simulink model "AW_test_bachup"  (R2015a)
settings: Solver=ode5  StartTime=0.0  StopTime=0.5  FixedStep=1e-5  MaxStep=5e-5  MinStep=1e-14  RelTol=1e-12  AbsTol=1e-12
values from neighbouring files (symbols this model uses):
  Ak = [-672.634870495 -2626.58972998 -46.1193303275 25.5793500122 108.891317034 -102.718752792 -245.794654799 -577.315326704 39.8827087547 153.58157137 60.36854216 -207.81122515 ... (144 elements, 12x12)]    [controller.mat]    (also in main_matlab.m = rlqg.A)
  Bk = [0.204306341627 1.11161335273 -0.324978673641 2.85402340631 -4.5813117605 2.97328839236 -0.174709893359 1.31662160979 2.94898293865 13.5567055967 -0.791381118401 0.0552385579013]    [controller.mat]    (also in main_matlab.m = rlqg.B)
  Ck = [534.788956442 909.016401092 107.069958755 -410.092366717 -1097.26369634 478.53061829 -894.210554118 460.341899649 -450.064931583 371.993181033 532.787728171 55.8162878584 ... (24 elements, 2x12)]    [controller.mat]    (also in main_matlab.m = rlqg.C)
  Dk = [0 0]    [controller.mat]    (also in main_matlab.m = rlqg.D)
  dumsys1 = ss(Ap+Bp*F,Bp*E,F,E-eye(size(E)))    [main_matlab.m]
  dumsys2 = ss(Ap+Bp*F,Bp*E,Cp+Dp*F,Dp*E)    [main_matlab.m]
undefined symbols (not defined in the file or in its folder): Af, Bf, Cf, Hf
settings Model: Creator=p4wp4w  LastModifiedBy=Ablah

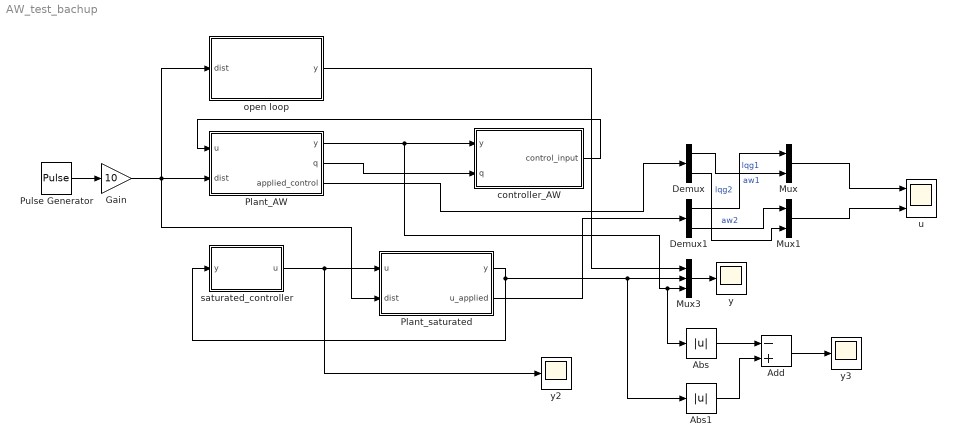
== system AW_test_bachup ==
  Abs : Abs
  Abs1 : Abs
  Add : Sum  Inputs=-+
  Demux : Demux  Outputs=2
  Demux1 : Demux  Outputs=2
  Gain : Gain  Gain=10
  Mux : Mux  Inputs=2
  Mux1 : Mux  Inputs=2
  Mux3 : Mux  Inputs=3
  Plant_AW : Subsystem
  Plant_saturated : Subsystem
  Pulse Generator : DiscretePulseGenerator  PulseType=Time based  Period=0.5  PulseWidth=10
  controller_AW : Subsystem
  open loop : Subsystem
  "saturated_controller " : Subsystem
  u : Scope  NumInputPorts=2
      settings: ShowLegends=on  YMin=-0.45~-0.2  YMax=0.2~0.125
  y : Scope
      settings: ShowLegends=on
  y2 : Scope
      settings: SaveName=ScopeData6
  y3 : Scope
      settings: ShowLegends=on  SaveName=ScopeData3
  wires:
  Plant_AW/1(y) -> Abs/1, Mux3/3, controller_AW/1(y)
  controller_AW/1("control_input ") -> Plant_AW/1(u)
  Pulse Generator/1 -> Gain/1
  Plant_saturated/1(y) -> Abs1/1, Mux3/2, "saturated_controller "/1(y)
  Demux1/1 -> Mux/1  "aw1"
  Demux/1 -> Mux/2  "lqg1"
  Demux1/2 -> Mux1/1  "aw2"
  Demux/2 -> Mux1/2  "lqg2"
  Mux/1 -> u/1
  Mux1/1 -> u/2
  Plant_saturated/2(u_applied) -> Demux1/1
  Gain/1 -> Plant_saturated/2(dist), open loop/1(dist), Plant_AW/2(dist)
  open loop/1(y) -> Mux3/1
  Mux3/1 -> y/1
  "saturated_controller "/1(u) -> y2/1, Plant_saturated/1(u)
  Abs/1 -> Add/1
  Abs1/1 -> Add/2
  Add/1 -> y3/1
  Plant_AW/2(q) -> controller_AW/2(q)
  Plant_AW/3(applied_control) -> Demux/1

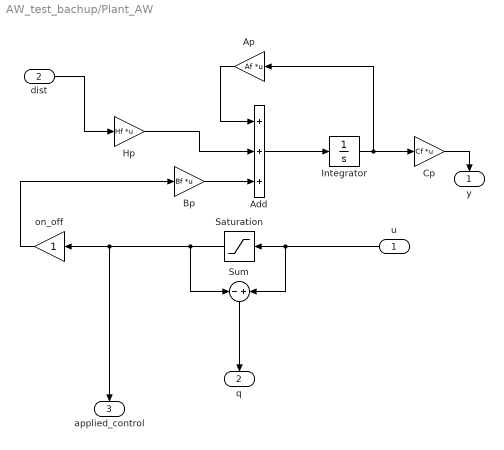
== system AW_test_bachup/Plant_AW ==
  u : Inport
  dist : Inport  Port=2
  Add : Sum  Inputs=+++
  Ap : Gain  Gain=Af  Multiplication=Matrix(K*u)
  Bp : Gain  Gain=Bf  Multiplication=Matrix(K*u)
  Cp : Gain  Gain=Cf  Multiplication=Matrix(K*u)
  Hp : Gain  Gain=Hf  Multiplication=Matrix(K*u)
  Integrator : Integrator
  Saturation : Saturate  UpperLimit=2  LowerLimit=-2
  Sum : Sum  Inputs=-|+
  on_off : Gain
  y : Outport
  q : Outport  Port=2
  applied_control : Outport  Port=3
  wires:
  Add/1 -> Integrator/1
  Cp/1 -> y/1
  Hp/1 -> Add/2
  on_off/1 -> Bp/1
  Integrator/1 -> Cp/1, Ap/1
  Ap/1 -> Add/1
  Bp/1 -> Add/3
  dist/1 -> Hp/1
  u/1 -> Sum/2, Saturation/1
  Saturation/1 -> Sum/1, on_off/1, applied_control/1
  Sum/1 -> q/1

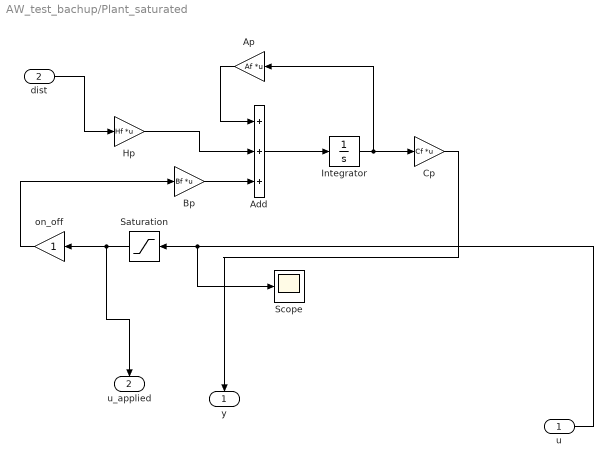
== system AW_test_bachup/Plant_saturated ==
  u : Inport
  dist : Inport  Port=2
  Add : Sum  Inputs=+++
  Ap : Gain  Gain=Af  Multiplication=Matrix(K*u)
  Bp : Gain  Gain=Bf  Multiplication=Matrix(K*u)
  Cp : Gain  Gain=Cf  Multiplication=Matrix(K*u)
  Hp : Gain  Gain=Hf  Multiplication=Matrix(K*u)
  Integrator : Integrator
  Saturation : Saturate  UpperLimit=2  LowerLimit=-2
  Scope : Scope
      settings: YMin=-10  YMax=10  SaveName=ScopeData2
  on_off : Gain
  y : Outport
  u_applied : Outport  Port=2
  wires:
  dist/1 -> Hp/1
  Bp/1 -> Add/3
  u/1 -> Scope/1, Saturation/1
  Ap/1 -> Add/1
  Saturation/1 -> u_applied/1, on_off/1
  Integrator/1 -> Ap/1, Cp/1
  on_off/1 -> Bp/1
  Hp/1 -> Add/2
  Cp/1 -> y/1
  Add/1 -> Integrator/1

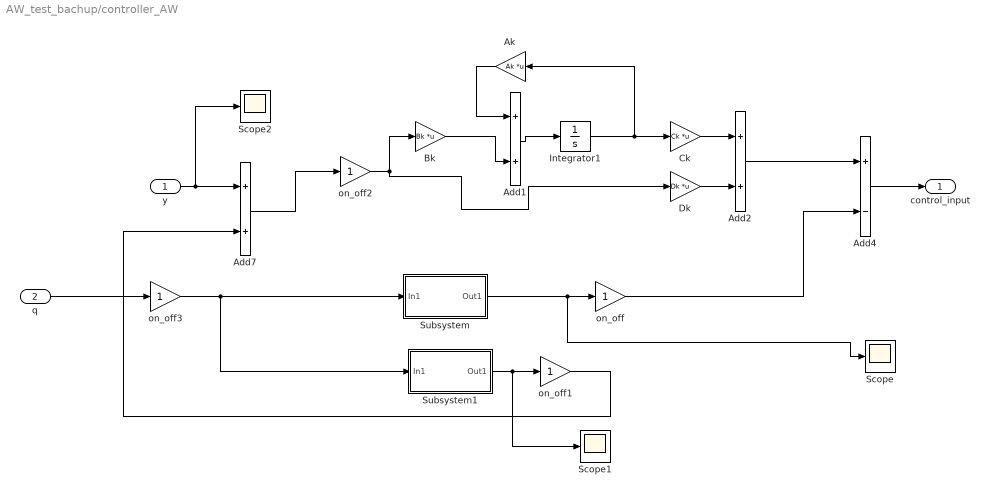
== system AW_test_bachup/controller_AW ==
  y : Inport
  q : Inport  Port=2
  Add1 : Sum
  Add2 : Sum
  Add4 : Sum  Inputs=+-
  Add7 : Sum
  Ak : Gain  Gain=Ak  Multiplication=Matrix(K*u)
  Bk : Gain  Gain=Bk  Multiplication=Matrix(K*u)
  Ck : Gain  Gain=Ck  Multiplication=Matrix(K*u)
  Dk : Gain  Gain=Dk  Multiplication=Matrix(K*u)
  Integrator1 : Integrator
  Scope : Scope
      settings: SaveName=ScopeData4
  Scope1 : Scope
      settings: SaveName=ScopeData5
  Scope2 : Scope
      settings: SaveName=ScopeData7
  Subsystem : Subsystem
  Subsystem1 : Subsystem
  on_off{,1..3} (4 alike) : Gain
  "control_input " : Outport
  wires:
  Ck/1 -> Add2/1
  Add1/1 -> Integrator1/1
  Ak/1 -> Add1/1
  Bk/1 -> Add1/2
  Integrator1/1 -> Ck/1, Ak/1
  Dk/1 -> Add2/2
  on_off2/1 -> Dk/1, Bk/1
  Add2/1 -> Add4/1
  Add4/1 -> "control_input "/1
  y/1 -> Scope2/1, Add7/1
  Add7/1 -> on_off2/1
  q/1 -> on_off3/1
  Subsystem/1(Out1) -> Scope/1, on_off/1
  Subsystem1/1(Out1) -> Scope1/1, on_off1/1
  on_off/1 -> Add4/2
  on_off1/1 -> Add7/2
  on_off3/1 -> Subsystem1/1(In1), Subsystem/1(In1)

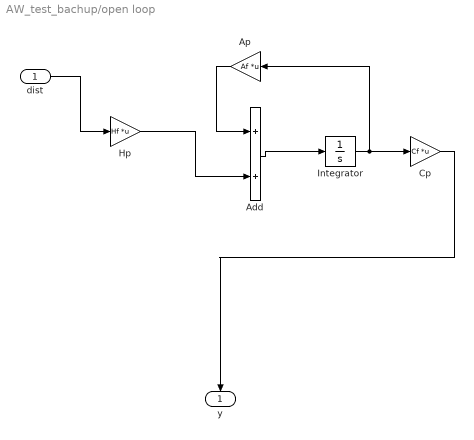
== system AW_test_bachup/open loop ==
  dist : Inport
  Add : Sum
  Ap : Gain  Gain=Af  Multiplication=Matrix(K*u)
  Cp : Gain  Gain=Cf  Multiplication=Matrix(K*u)
  Hp : Gain  Gain=Hf  Multiplication=Matrix(K*u)
  Integrator : Integrator
  y : Outport
  wires:
  dist/1 -> Hp/1
  Ap/1 -> Add/1
  Integrator/1 -> Ap/1, Cp/1
  Hp/1 -> Add/2
  Cp/1 -> y/1
  Add/1 -> Integrator/1

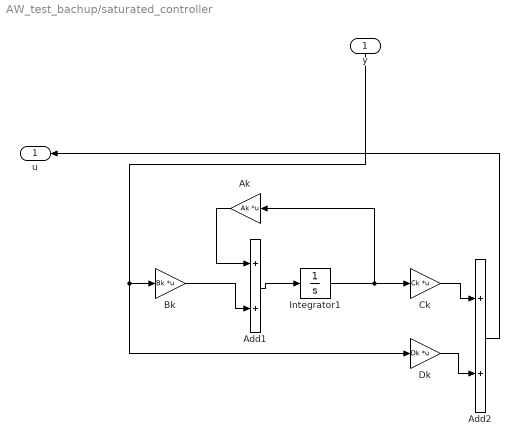
== system AW_test_bachup/saturated_controller  ==
  y : Inport
  Add1 : Sum
  Add2 : Sum
  Ak : Gain  Gain=Ak  Multiplication=Matrix(K*u)
  Bk : Gain  Gain=Bk  Multiplication=Matrix(K*u)
  Ck : Gain  Gain=Ck  Multiplication=Matrix(K*u)
  Dk : Gain  Gain=Dk  Multiplication=Matrix(K*u)
  Integrator1 : Integrator
  u : Outport
  wires:
  Bk/1 -> Add1/2
  Add1/1 -> Integrator1/1
  Ck/1 -> Add2/1
  Dk/1 -> Add2/2
  Integrator1/1 -> Ck/1, Ak/1
  Add2/1 -> u/1
  Ak/1 -> Add1/1
  y/1 -> Bk/1, Dk/1

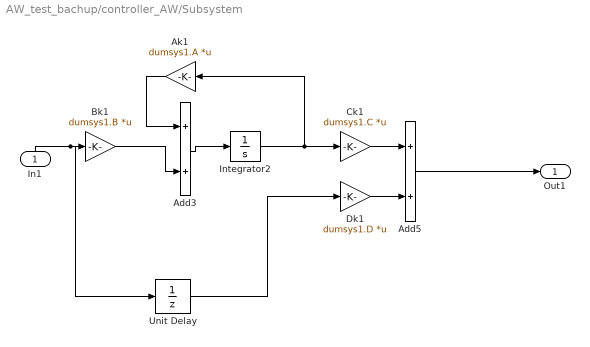
== system AW_test_bachup/controller_AW/Subsystem ==
  In1 : Inport
  Add3 : Sum
  Add5 : Sum
  Ak1 : Gain  Gain=dumsys1.A  Multiplication=Matrix(K*u)
  Bk1 : Gain  Gain=dumsys1.B  Multiplication=Matrix(K*u)
  Ck1 : Gain  Gain=dumsys1.C  Multiplication=Matrix(K*u)
  Dk1 : Gain  Gain=dumsys1.D  Multiplication=Matrix(K*u)
  Integrator2 : Integrator
  Unit Delay : UnitDelay  SampleTime=-1
  Out1 : Outport
  wires:
  Bk1/1 -> Add3/2
  In1/1 -> Unit Delay/1, Bk1/1
  Ak1/1 -> Add3/1
  Add3/1 -> Integrator2/1
  Ck1/1 -> Add5/1
  Dk1/1 -> Add5/2
  Add5/1 -> Out1/1
  Integrator2/1 -> Ak1/1, Ck1/1
  Unit Delay/1 -> Dk1/1

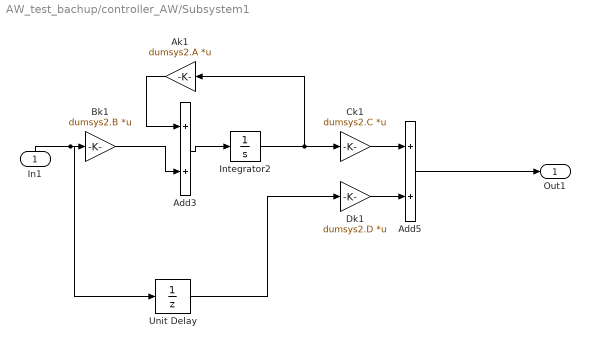
== system AW_test_bachup/controller_AW/Subsystem1 ==
  In1 : Inport
  Add3 : Sum
  Add5 : Sum
  Ak1 : Gain  Gain=dumsys2.A  Multiplication=Matrix(K*u)
  Bk1 : Gain  Gain=dumsys2.B  Multiplication=Matrix(K*u)
  Ck1 : Gain  Gain=dumsys2.C  Multiplication=Matrix(K*u)
  Dk1 : Gain  Gain=dumsys2.D  Multiplication=Matrix(K*u)
  Integrator2 : Integrator
  Unit Delay : UnitDelay  SampleTime=-1
  Out1 : Outport
  wires:
  Unit Delay/1 -> Dk1/1
  Integrator2/1 -> Ck1/1, Ak1/1
  Add5/1 -> Out1/1
  Dk1/1 -> Add5/2
  Ck1/1 -> Add5/1
  Add3/1 -> Integrator2/1
  Ak1/1 -> Add3/1
  In1/1 -> Bk1/1, Unit Delay/1
  Bk1/1 -> Add3/2
